simulink model "engine"  (R2019b)
settings: Solver=VariableStepAuto  StartTime=0.0  StopTime=9  MaxStep=1e-2  RelTol=1e-3
libraries: cstblocks x18, simulink x1
(part 2 of 2)

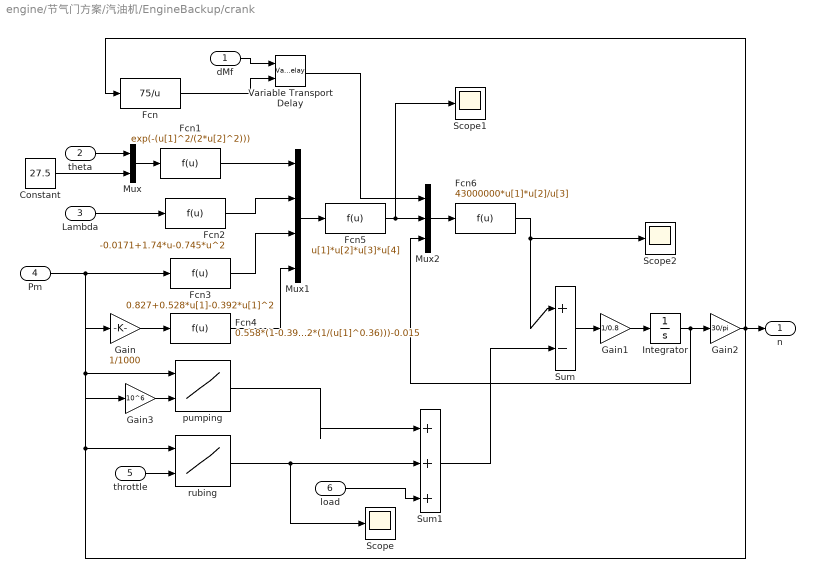
== system engine/节气门方案/汽油机/EngineBackup/crank ==
  dMf : Inport
  theta : Inport  Port=2
  Lambda : Inport  Port=3
  Pm : Inport  Port=4
  throttle : Inport  Port=5
  load : Inport  Port=6
  Constant : Constant  Value=27.5
  Fcn : Fcn  Expr=75/u
  Fcn1 : Fcn  Expr=exp(-(u[1]^2/(2*u[2]^2)))
  Fcn2 : Fcn  Expr=-0.0171+1.74*u-0.745*u^2
  Fcn3 : Fcn  Expr=0.827+0.528*u[1]-0.392*u[1]^2
  Fcn4 : Fcn  Expr=0.558*(1-0.392*(1/(u[1]^0.36)))-0.015
  Fcn5 : Fcn  Expr=u[1]*u[2]*u[3]*u[4]
  Fcn6 : Fcn  Expr=43000000*u[1]*u[2]/u[3]
  Gain : Gain  Gain=1/1000  SaturateOnIntegerOverflow=on  OutDataTypeStr=Inherit: Same as input  ParamDataTypeStr=Inherit: Same as input
  Gain1 : Gain  Gain=1/0.8  SaturateOnIntegerOverflow=on  OutDataTypeStr=Inherit: Same as input  ParamDataTypeStr=Inherit: Same as input
  Gain2 : Gain  Gain=30/pi  SaturateOnIntegerOverflow=on  OutDataTypeStr=Inherit: Same as input  ParamDataTypeStr=Inherit: Same as input
  Gain3 : Gain  Gain=10^6  SaturateOnIntegerOverflow=on  OutDataTypeStr=Inherit: Same as input  ParamDataTypeStr=Inherit: Same as input
  Integrator : Integrator  InitialCondition=349
  Mux : Mux  Inputs=2
  Mux1 : Mux
  Mux2 : Mux  Inputs=3
  Scope : Scope
  Scope1 : Scope
  Scope2 : Scope
  Sum : Sum  Inputs=|+-  SaturateOnIntegerOverflow=on
  Sum1 : Sum  Inputs=|+++  SaturateOnIntegerOverflow=on
  Variable Transport Delay : VariableTransportDelay  MaximumDelay=10
  pumping : Lookup2D  RowIndex=[800 1600 2400 3200 4000 4800 5600 6400]  ColumnIndex=[20000 30000 40000 50000 60000 70000 80000 90000 100000]  Table=[19.6 17.64 15.68 15.68 13.72 11.76 7.84 5.88 3.92;21.56 19.6 17.64 15.68 13.72 11.76 9.8 7.84 3.92;23.52 21.56 19.6 17.64 15.68 13.72 11.76 9.8 7.84;23.52 23.52 19.6 19.6 15.68 15.68 15.68 15.68 13.72;23.52 23.52 23.52 21.56 21.56 21.56 19.6 19.6 19.6;23.52 23.52 23.52 23.52 23.52 25.48 25.48 25.48 25.48;23.52 25.48 25.48 27.44 29.4 31.36 33.32 33.32 35.28;23.52 25.48 27.44 29.4 29.4 31.36 35.28 37.24 39.2]  SaturateOnIntegerOverflow=on
  rubing : Lookup2D  RowIndex=[800 1600 2400 3200 4000 4800 5600 6400]  ColumnIndex=[8 20 32 44 56 68 80 92 104 116]  Table=[31.36 29.4 25.48 23.52 21.56 17.64 15.68 13.72 13.72 13.72;31.36 29.4 25.48 23.52 21.56 17.64 15.68 13.72 13.72 13.72;33.32 29.4 27.44 25.48 21.56 19.6 17.64 15.68 15.68 15.68;33.32 31.36 27.44 25.48 23.52 19.6 17.64 15.68 15.68 15.68;35.28 33.32 29.4 27.44 25.48 21.56 19.6 17.64 17.64 17.64;39.2 37.24 33.32 31.36 29.4 25.48 23.52 21.56 21.56 21.56;45.08 41.16 39.2 37.24 33.32 31.36 29.4 27.44 27.44 27.44;52.92 49 45.08 43.12 41.16 37.24 35.28 33.32 33.32 33.32]  SaturateOnIntegerOverflow=on
  n : Outport
  wires:
  Integrator/1 -> Mux2/3, Gain2/1
  Gain3/1 -> pumping/2
  Sum1/1 -> Sum/2
  load/1 -> Sum1/3
  rubing/1 -> Scope/1, Sum1/2
  pumping/1 -> Sum1/1
  Gain2/1 -> pumping/1, Gain/1, rubing/1, Fcn/1, n/1
  Gain1/1 -> Integrator/1
  Sum/1 -> Gain1/1
  Fcn6/1 -> Scope2/1, Sum/1
  Mux2/1 -> Fcn6/1
  Variable Transport Delay/1 -> Mux2/1
  Fcn5/1 -> Mux2/2, Scope1/1
  Mux1/1 -> Fcn5/1
  throttle/1 -> rubing/2
  Pm/1 -> Fcn3/1, Gain3/1
  Gain/1 -> Fcn4/1
  Fcn4/1 -> Mux1/4
  Fcn3/1 -> Mux1/3
  Fcn2/1 -> Mux1/2
  Fcn1/1 -> Mux1/1
  Lambda/1 -> Fcn2/1
  Mux/1 -> Fcn1/1
  Constant/1 -> Mux/2
  theta/1 -> Mux/1
  Fcn/1 -> Variable Transport Delay/2
  dMf/1 -> Variable Transport Delay/1

== system engine/节气门方案/汽油机/EngineBackup/fuel ==
  a_throttle : Inport
  n : Inport  Port=2
  dMfu : Inport  Port=3
  Subsystem : Subsystem
  Subsystem1 : Subsystem
  dMf : Outport
  wires:
  Subsystem/1(X) -> Subsystem1/2(X)
  Subsystem/2(tau) -> Subsystem1/3(tau)
  Subsystem/3(dMfi) -> Subsystem1/1(dMfi)
  Subsystem1/1(dMf) -> dMf/1
  dMfu/1 -> Subsystem/3(dMfu)
  n/1 -> Subsystem/2(n)
  a_throttle/1 -> Subsystem/1(a_throttle)

== system engine/节气门方案/汽油机/动力输出子模型/摩擦阻力 ==
  Rpm : Inport
  Gain : Gain  Gain=1000
  Sum : Sum  Inputs=|++
  其它机械阻力 : Lookup_n-D  NumberOfTableDimensions=1  BreakpointsForDimension1=[-1000,0,1000,2000,3000,4000,5000,6000,7000]  BreakpointsForDimension2=[1:3]  Table=[-10,0,2.4757,5.0728,8.568,13.3738,18.9078,26.4806,35]  InternalRulePriority=Speed  RndMeth=Simplest  InputSameDT=on
  最大静摩擦 : Saturate  UpperLimit=10  LowerLimit=-10
  摩擦阻力 : Outport
  wires:
  其它机械阻力/1 -> Sum/2
  Sum/1 -> 摩擦阻力/1
  Rpm/1 -> Gain/1, 其它机械阻力/1
  Gain/1 -> 最大静摩擦/1
  最大静摩擦/1 -> Sum/1  "摩擦阻力"

== system engine/节气门方案/汽油机/动力输出子模型/泵气损失 ==
  Pman-kPa : Inport
  rpm : Inport  Port=2
  Lookup::泵气损失 : Lookup_n-D  NumberOfTableDimensions=1  BreakpointsForDimension1=[0,10,20,50,70,90,110,120]  BreakpointsForDimension2=[-250,0,250,500,750,1000,2000,3000,4000,5000,6000,7000]  Table=[99.84,58.6364,37.4242,19.8485,13.1818,9.2424,7.1212,6.5152]  DiagnosticForOutOfRangeInput=Warning  InternalRulePriority=Speed  RndMeth=Simplest  InputSameDT=on
  Product : Product
  泵气损失转速系数 : Gain  Gain=1/1000
  泵气损失 : Outport
  wires:
  rpm/1 -> 泵气损失转速系数/1
  Product/1 -> 泵气损失/1
  Pman-kPa/1 -> Lookup::泵气损失/1
  Lookup::泵气损失/1 -> Product/1
  泵气损失转速系数/1 -> Product/2

== system engine/节气门方案/汽油机/喷油控制、燃油模型/喷油控制算法 ==
  note: dMfv: 需要的燃油蒸汽流量
      | X:燃油喷射沉积比例
  note: dMfu: 通过当前发动机进气量和理论空燃比计算的气缸进油量
  X : Inport
  tau : Inport  Port=2
  dMfu : Inport  Port=3
  Mux : Mux  Inputs=2
  Sum : Sum  Inputs=|+-  SaturateOnIntegerOverflow=on
  由dMfv算dMfi : Fcn  Expr=u[2]/(1-u[1])
  计算油膜蒸发速率:dMff : Subsystem
  dMfi : Outport
  wires:
  计算油膜蒸发速率:dMff/1(dMff) -> Sum/2
  tau/1 -> 计算油膜蒸发速率:dMff/1(tau)
  X/1 -> Mux/1, 计算油膜蒸发速率:dMff/2(X)
  Mux/1 -> 由dMfv算dMfi/1
  由dMfv算dMfi/1 -> 计算油膜蒸发速率:dMff/3(dMfi), dMfi/1  "dMfi"
  Sum/1 -> Mux/2  "dMfv"
  dMfu/1 -> Sum/1

== system engine/节气门方案/汽油机/喷油控制、燃油模型/查表得当前X和tau ==
  throttle : Inport
  n : Inport  Port=2
  Look-Up Table (2-D) : Lookup2D  RowIndex=[0.1 0.2 0.3 0.4 0.5 0.6 0.7 0.8]  ColumnIndex=[1500 2000 2500 3000 4000 5000 6000]  Table=[0.842 0.852 0.852 0.824 0.824 0.842 0.85;0.814 0.847 0.837 0.853 0.85 0.86 0.84;0.838 0.836 0.845 0.856 0.84 0.82 0.86;0.836 0.815 0.865 0.842 0.82 0.87 0.84;0.845 0.824 0.828 0.824 0.85 0.83 0.84;0.841 0.822 0.813 0.832 0.823 0.832 0.845;0.832 0.821 0.841 0.825 0.820 0.832 0.841;0.815 0.808 0.826 0.832 0.815 0.82 0.83]  SaturateOnIntegerOverflow=on
  Look-Up Table (2-D)1 : Lookup2D  RowIndex=[0.1 0.2 0.3 0.4 0.5 0.6 0.7 0.8]  ColumnIndex=[1500 2000 2500 3000 4000 5000 6000]  Table=[0.303 0.238 0.174 0.127 0.125 0.124 0.12;0.335 0.241 0.184 0.131 0.13 0.129 0.12;0.365 0.254 0.195 0.147 0.145 0.125 0.12; 0.374 0.275 0.208 0.152 0.15 0.14 0.13;0.395 0.305 0.216 0.163 0.16 0.15 0.14;0.425 0.336 0.235 0.175 0.170 0.160 0.155;0.438 0.351 0.257 0.182 0.171 0.16 0.54;0.446 0.354 0.262 0.194 0.18 0.175 0.16]  SaturateOnIntegerOverflow=on
  X : Outport
  tau : Outport  Port=2
  wires:
  n/1 -> Look-Up Table (2-D)1/2, Look-Up Table (2-D)/2
  Look-Up Table (2-D)/1 -> X/1
  Look-Up Table (2-D)1/1 -> tau/1
  throttle/1 -> Look-Up Table (2-D)1/1, Look-Up Table (2-D)/1

== system engine/节气门方案/汽油机/喷油控制、燃油模型/燃油模型 ==
  X : Inport
  tau : Inport  Port=2
  dMfi : Inport  Port=3
  1-X : Fcn  Expr=u[1]*(1-u[2])
  1/tau : Math  Operator=reciprocal  SaturateOnIntegerOverflow=on
  Fcn : Fcn  Expr=u[1]*u[2]
  Fcn1 : Fcn  Expr=u[1]*u[2]
  Integrator : Integrator
  Mux : Mux  Inputs=2
  Mux1 : Mux  Inputs=2
  Mux2 : Mux  Inputs=2
  Sum : Sum  Inputs=|++  SaturateOnIntegerOverflow=on
  Sum1 : Sum  Inputs=|+-  SaturateOnIntegerOverflow=on
  X1 : Fcn  Expr=u[1]*u[2]
  dMf : Outport
  wires:
  dMfi/1 -> Mux/1
  X/1 -> Mux/2
  tau/1 -> 1/tau/1
  Sum/1 -> dMf/1
  Fcn1/1 -> Sum1/2
  Mux2/1 -> Fcn1/1
  Integrator/1 -> Sum/2, Mux2/1
  Sum1/1 -> Integrator/1
  Fcn/1 -> Sum1/1
  1-X/1 -> Sum/1
  Mux1/1 -> Fcn/1
  1/tau/1 -> Mux2/2, Mux1/2
  X1/1 -> Mux1/1  "X*dMfi"
  Mux/1 -> X1/1, 1-X/1

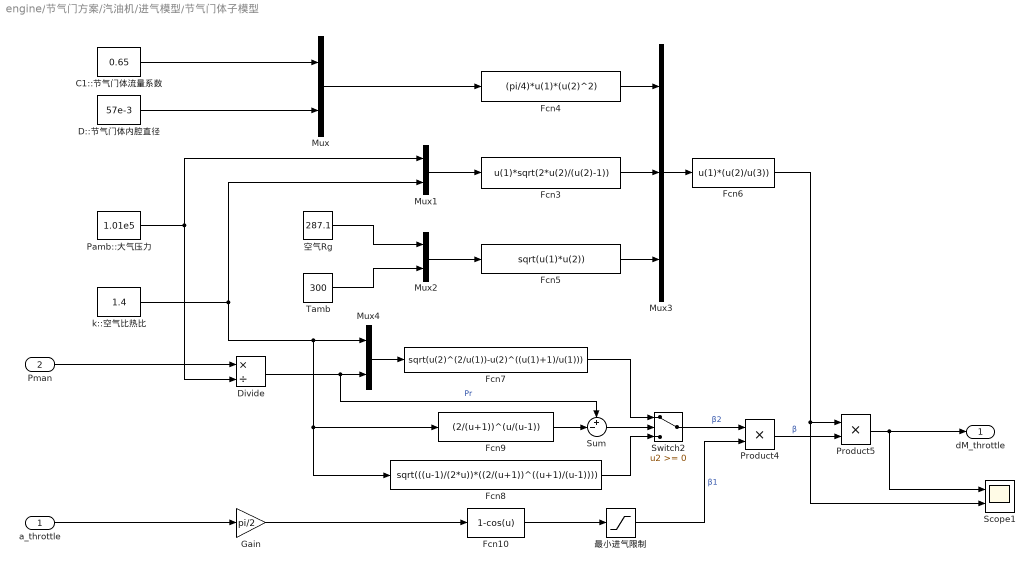
== system engine/节气门方案/汽油机/进气模型/节气门体子模型 ==
  a_throttle : Inport
  Pman : Inport  Port=2
  C1::节气门体流量系数 : Constant  Value=0.65
  D::节气门体内腔直径 : Constant  Value=57e-3
  Divide : Product  Inputs=*/
  Fcn10 : Fcn  Expr=1-cos(u)
  Fcn3 : Fcn  Expr=u(1)*sqrt(2*u(2)/(u(2)-1))
  Fcn4 : Fcn  Expr=(pi/4)*u(1)*(u(2)^2)
  Fcn5 : Fcn  Expr=sqrt(u(1)*u(2))
  Fcn6 : Fcn  Expr=u(1)*(u(2)/u(3))
  Fcn7 : Fcn  Expr=sqrt(u(2)^(2/u(1))-u(2)^((u(1)+1)/u(1)))
  Fcn8 : Fcn  Expr=sqrt(((u-1)/(2*u))*((2/(u+1))^((u+1)/(u-1))))
  Fcn9 : Fcn  Expr=(2/(u+1))^(u/(u-1))
  Gain : Gain  Gain=pi/2
  Mux{,1..2,4} (4 alike) : Mux  Inputs=2
  Mux3 : Mux  Inputs=3
  Pamb::大气压力 : Constant  Value=1.01e5
  Product4 : Product
  Product5 : Product
  Scope1 : Scope  NumInputPorts=2
  Sum : Sum  Inputs=+-|
  Switch2 : Switch  SaturateOnIntegerOverflow=on
  Tamb : Constant  Value=300
  k::空气比热比 : Constant  Value=1.4
  最小进气限制 : Saturate  UpperLimit=1  LowerLimit=0.01
  空气Rg : Constant  Value=287.1
  dM_throttle : Outport
  wires:
  最小进气限制/1 -> Product4/2  "β1"
  Product5/1 -> Scope1/1, dM_throttle/1
  Fcn6/1 -> Product5/1, Scope1/2
  Product4/1 -> Product5/2  "β"
  Gain/1 -> Fcn10/1
  Fcn10/1 -> 最小进气限制/1
  a_throttle/1 -> Gain/1
  Switch2/1 -> Product4/1  "β2"
  Fcn7/1 -> Switch2/1
  Sum/1 -> Switch2/2
  Fcn9/1 -> Sum/2
  Mux4/1 -> Fcn7/1
  Divide/1 -> Mux4/2, Sum/1  "Pr"
  Mux3/1 -> Fcn6/1
  Fcn4/1 -> Mux3/1
  Fcn5/1 -> Mux3/3
  Fcn3/1 -> Mux3/2
  Mux2/1 -> Fcn5/1
  空气Rg/1 -> Mux2/1
  Tamb/1 -> Mux2/2
  Mux1/1 -> Fcn3/1
  k::空气比热比/1 -> Mux4/1, Fcn8/1, Fcn9/1, Mux1/2
  Pamb::大气压力/1 -> Divide/2, Mux1/1
  Mux/1 -> Fcn4/1
  D::节气门体内腔直径/1 -> Mux/2
  C1::节气门体流量系数/1 -> Mux/1
  Fcn8/1 -> Switch2/3
  Pman/1 -> Divide/1

== system engine/节气门方案/汽油机/进气模型/进气歧管子模型 ==
  dM_throttle : Inport
  dM_air_engine : Inport  Port=2
  Gain : Gain  Gain=0.5
  Integrator : Integrator
  Pamb::大气压力 : Constant  Value=1.01e5
  RTm/Vm : Gain  Gain=(287.1*323)/(1.875*(10^(-3)))  SaturateOnIntegerOverflow=on  OutDataTypeStr=Inherit: Same as input  ParamDataTypeStr=Inherit: Same as input
  Sum : Sum  Inputs=|+-  SaturateOnIntegerOverflow=on
  Sum1 : Sum  Inputs=|++
  Pman : Outport
  wires:
  Gain/1 -> Sum1/2
  Pamb::大气压力/1 -> Gain/1
  Sum1/1 -> Pman/1
  dM_throttle/1 -> Sum/1
  dM_air_engine/1 -> Sum/2
  RTm/Vm/1 -> Integrator/1
  Integrator/1 -> Sum1/1
  Sum/1 -> RTm/Vm/1

== system engine/节气门方案/汽油机/进气模型/进气门口模型 ==
  note: Map: 离开进气管，进入燃烧室的空气质量流动速率
  note: Map = n*Vd*η-vol*Pman/(120*R*Tman)
  Pman : Inport
  n : Inport  Port=2
  120R : Gain  Gain=120*287.1  SaturateOnIntegerOverflow=on  OutDataTypeStr=Inherit: Same as input  ParamDataTypeStr=Inherit: Same as input
  Look-Up Table: η-vol : Lookup2D  RowIndex=[40000 50000 65000 80000 90000 95000]  ColumnIndex=[1000 1500 2000 3000 3500 4000 4500 5000]  Table=[0.431 0.5172 0.5532 0.6159 0.5862 0.5847 0.5232 0.4465;0.5705 0.6442 0.6558 0.7246 0.6668 0.6728 0.6235 0.5869;0.6559 0.7401 0.7581 0.7887 0.7638 0.762 0.7321 0.6658;0.7155 0.8231 0.8345 0.8446 0.8279 0.8416 0.8165 0.7365;0.8115 0.8741 0.8636 0.8924 0.8572 0.8752 0.8632 0.8254;0.8621 0.9053 0.9054 0.937 0.904 0.909 0.8865 0.8569]  SaturateOnIntegerOverflow=on
  Product : Product  SaturateOnIntegerOverflow=on  OutDataTypeStr=Inherit: Same as first input
  Product1 : Product  Inputs=***/  SaturateOnIntegerOverflow=on  OutDataTypeStr=Inherit: Same as first input
  Tman : Constant  Value=323
  Vd : Constant  Value=1.5*(10^-3)
  Map : Outport
  wires:
  Pman/1 -> Look-Up Table: η-vol/1, Product/1
  n/1 -> Look-Up Table: η-vol/2, Product/2
  Product/1 -> Product1/1
  Vd/1 -> Product1/2
  Look-Up Table: η-vol/1 -> Product1/3  "η-vol"
  Tman/1 -> 120R/1
  120R/1 -> Product1/4
  Product1/1 -> Map/1  "Map"

== system engine/节气门方案/转速-功率标定/Subsystem1/LPF ==
  Signal : Inport
  Constant2 : Constant  Value=Frq
  Gain : Gain  Gain=2*pi
  d_Smp_LPF6 : cstblocks/Linear Parameter Varying/Varying Lowpass Filter  N=Order
      settings: SourceProductName=Control System Toolbox
  Output : Outport
  wires:
  d_Smp_LPF6/1 -> Output/1  "Is"
  Constant2/1 -> Gain/1
  Signal/1 -> d_Smp_LPF6/1
  Gain/1 -> d_Smp_LPF6/2

== system engine/节气门方案/转速闭环/微分/微分滤波1 ==
  Signal : Inport
  Constant2 : Constant  Value=Frq
  Gain : Gain  Gain=2*pi
  d_Smp_LPF6 : cstblocks/Linear Parameter Varying/Varying Lowpass Filter  N=Order
      settings: SourceProductName=Control System Toolbox
  Output : Outport
  wires:
  d_Smp_LPF6/1 -> Output/1  "Is"
  Constant2/1 -> Gain/1
  Signal/1 -> d_Smp_LPF6/1
  Gain/1 -> d_Smp_LPF6/2

== system engine/节气门方案/转速闭环/积分控制/Subsystem ==
  dErr : Inport
  Err : Inport  Port=2
  Abs : Abs
  Constant10 : Constant
  Constant3 : Constant  Value=0
  Constant4 : Constant
  Memory2 : Memory
  Product : Product
  Switch1 : Switch  Criteria=u2 > Threshold  Threshold=dRPM
  Switch6 : Switch  Criteria=u2 > Threshold
  启动积分 : Outport
  wires:
  Switch1/1 -> 启动积分/1
  Err/1 -> Product/2
  Switch6/1 -> Switch1/1
  Product/1 -> Memory2/1
  Constant3/1 -> Switch6/3
  Abs/1 -> Switch1/2
  Constant4/1 -> Switch1/3
  Constant10/1 -> Switch6/1
  dErr/1 -> Abs/1, Product/1
  Memory2/1 -> Switch6/2

== system engine/节气门方案/转速闭环/积分控制/输出达到正限幅时积分不再增大 ==
  Err : Inport
  Out : Inport  Port=2
  Constant : Constant  Value=Trq_p
  Constant2 : Constant
  Constant5 : Constant  Value=0
  Constant6 : Constant
  Sum2 : Sum  Inputs=-+|
  Switch2 : Switch  Criteria=u2 > Threshold
  Switch3 : Switch  Criteria=u2 > Threshold
  启动积分 : Outport
  wires:
  Err/1 -> Switch2/2
  Switch3/1 -> Switch2/1
  Constant/1 -> Sum2/1
  Constant2/1 -> Switch2/3
  Constant6/1 -> Switch3/3
  Out/1 -> Sum2/2
  Sum2/1 -> Switch3/2
  Switch2/1 -> 启动积分/1
  Constant5/1 -> Switch3/1

== system engine/节气门方案/转速闭环/积分控制/输出达到负限幅时积分不再减小 ==
  Err : Inport
  Out : Inport  Port=2
  Constant1 : Constant
  Constant7 : Constant  Value=0
  Constant8 : Constant
  Constant9 : Constant  Value=-Trq_n
  Sum3 : Sum  Inputs=+-|
  Switch4 : Switch  Criteria=u2 > Threshold
  Switch5 : Switch  Criteria=u2 > Threshold
  启动积分 : Outport
  wires:
  Constant8/1 -> Switch5/3
  Switch4/1 -> 启动积分/1
  Constant7/1 -> Switch5/1
  Constant9/1 -> Sum3/1
  Constant1/1 -> Switch4/1
  Err/1 -> Switch4/2
  Out/1 -> Sum3/2
  Switch5/1 -> Switch4/3
  Sum3/1 -> Switch5/2

== system engine/转速方案/功率闭环/微分/微分滤波1 ==
  Signal : Inport
  Constant2 : Constant  Value=Frq
  Gain : Gain  Gain=2*pi
  d_Smp_LPF6 : cstblocks/Linear Parameter Varying/Varying Lowpass Filter  N=Order
      settings: SourceProductName=Control System Toolbox
  Output : Outport
  wires:
  d_Smp_LPF6/1 -> Output/1  "Is"
  Constant2/1 -> Gain/1
  Signal/1 -> d_Smp_LPF6/1
  Gain/1 -> d_Smp_LPF6/2

== system engine/转速方案/功率闭环/积分控制/Subsystem ==
  dErr : Inport
  Err : Inport  Port=2
  Abs : Abs
  Constant10 : Constant
  Constant3 : Constant  Value=0
  Constant4 : Constant
  Memory2 : Memory
  Product : Product
  Switch1 : Switch  Criteria=u2 > Threshold  Threshold=dPWR
  Switch6 : Switch  Criteria=u2 > Threshold
  启动积分 : Outport
  wires:
  Switch1/1 -> 启动积分/1
  Err/1 -> Product/2
  Switch6/1 -> Switch1/1
  Product/1 -> Memory2/1
  Constant3/1 -> Switch6/3
  Abs/1 -> Switch1/2
  Constant4/1 -> Switch1/3
  Constant10/1 -> Switch6/1
  dErr/1 -> Abs/1, Product/1
  Memory2/1 -> Switch6/2

== system engine/转速方案/功率闭环/积分控制/输出达到正限幅时积分不再增大 ==
  Err : Inport
  Out : Inport  Port=2
  Constant : Constant  Value=Acc_p
  Constant2 : Constant
  Constant5 : Constant  Value=0
  Constant6 : Constant
  Sum2 : Sum  Inputs=-+|
  Switch2 : Switch  Criteria=u2 > Threshold
  Switch3 : Switch  Criteria=u2 > Threshold
  启动积分 : Outport
  wires:
  Err/1 -> Switch2/2
  Switch3/1 -> Switch2/1
  Constant/1 -> Sum2/1
  Constant2/1 -> Switch2/3
  Constant6/1 -> Switch3/3
  Out/1 -> Sum2/2
  Sum2/1 -> Switch3/2
  Switch2/1 -> 启动积分/1
  Constant5/1 -> Switch3/1

== system engine/转速方案/功率闭环/积分控制/输出达到负限幅时积分不再减小 ==
  Err : Inport
  Out : Inport  Port=2
  Constant1 : Constant
  Constant7 : Constant  Value=0
  Constant8 : Constant
  Constant9 : Constant  Value=-Acc_n
  Sum3 : Sum  Inputs=+-|
  Switch4 : Switch  Criteria=u2 > Threshold
  Switch5 : Switch  Criteria=u2 > Threshold
  启动积分 : Outport
  wires:
  Constant8/1 -> Switch5/3
  Switch4/1 -> 启动积分/1
  Constant7/1 -> Switch5/1
  Constant9/1 -> Sum3/1
  Constant1/1 -> Switch4/1
  Err/1 -> Switch4/2
  Out/1 -> Sum3/2
  Switch5/1 -> Switch4/3
  Sum3/1 -> Switch5/2

== system engine/转速方案/汽油机/EngineBackup/air model ==
  n : Inport
  a_throttle : Inport  Port=2
  Gain : Gain  Gain=1/14.7  SaturateOnIntegerOverflow=on  OutDataTypeStr=Inherit: Same as input  ParamDataTypeStr=Inherit: Same as input
  Subsystem : Subsystem
  Subsystem1 : Subsystem
  Subsystem2 : Subsystem
  "dM_air_engine " : Outport
  dMfu : Outport  Port=2
  Pm_pa : Outport  Port=3
  wires:
  n/1 -> Subsystem/2(n)
  Subsystem/1(dM_air_engine) -> "dM_air_engine "/1, Gain/1, Subsystem2/2(dM_air_engine)
  Gain/1 -> dMfu/1
  a_throttle/1 -> Subsystem1/1(a_throttle)
  Subsystem2/1(Pm_pa) -> Pm_pa/1, Subsystem1/2(Pm_pa), Subsystem/1(Pm)
  Subsystem1/1(dM_throttle) -> Subsystem2/1(dM_throttle)

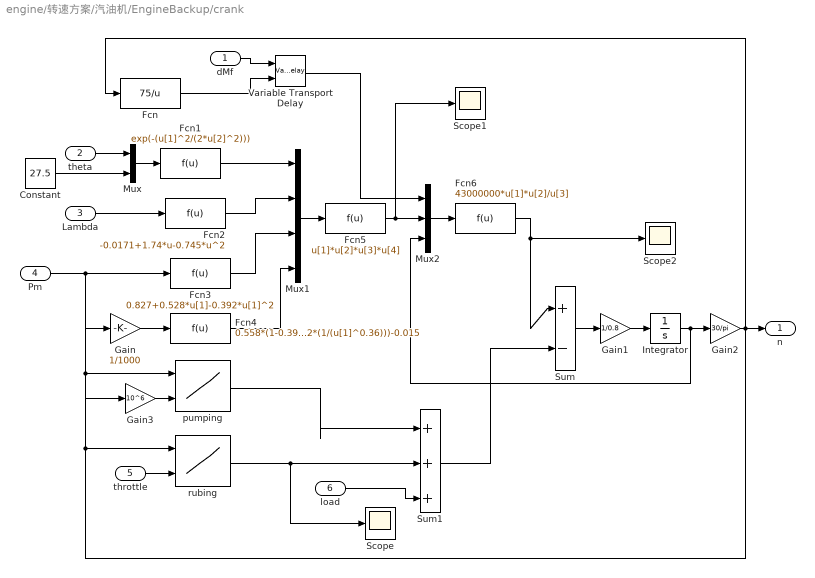
== system engine/转速方案/汽油机/EngineBackup/crank ==
  dMf : Inport
  theta : Inport  Port=2
  Lambda : Inport  Port=3
  Pm : Inport  Port=4
  throttle : Inport  Port=5
  load : Inport  Port=6
  Constant : Constant  Value=27.5
  Fcn : Fcn  Expr=75/u
  Fcn1 : Fcn  Expr=exp(-(u[1]^2/(2*u[2]^2)))
  Fcn2 : Fcn  Expr=-0.0171+1.74*u-0.745*u^2
  Fcn3 : Fcn  Expr=0.827+0.528*u[1]-0.392*u[1]^2
  Fcn4 : Fcn  Expr=0.558*(1-0.392*(1/(u[1]^0.36)))-0.015
  Fcn5 : Fcn  Expr=u[1]*u[2]*u[3]*u[4]
  Fcn6 : Fcn  Expr=43000000*u[1]*u[2]/u[3]
  Gain : Gain  Gain=1/1000  SaturateOnIntegerOverflow=on  OutDataTypeStr=Inherit: Same as input  ParamDataTypeStr=Inherit: Same as input
  Gain1 : Gain  Gain=1/0.8  SaturateOnIntegerOverflow=on  OutDataTypeStr=Inherit: Same as input  ParamDataTypeStr=Inherit: Same as input
  Gain2 : Gain  Gain=30/pi  SaturateOnIntegerOverflow=on  OutDataTypeStr=Inherit: Same as input  ParamDataTypeStr=Inherit: Same as input
  Gain3 : Gain  Gain=10^6  SaturateOnIntegerOverflow=on  OutDataTypeStr=Inherit: Same as input  ParamDataTypeStr=Inherit: Same as input
  Integrator : Integrator  InitialCondition=349
  Mux : Mux  Inputs=2
  Mux1 : Mux
  Mux2 : Mux  Inputs=3
  Scope : Scope
  Scope1 : Scope
  Scope2 : Scope
  Sum : Sum  Inputs=|+-  SaturateOnIntegerOverflow=on
  Sum1 : Sum  Inputs=|+++  SaturateOnIntegerOverflow=on
  Variable Transport Delay : VariableTransportDelay  MaximumDelay=10
  pumping : Lookup2D  RowIndex=[800 1600 2400 3200 4000 4800 5600 6400]  ColumnIndex=[20000 30000 40000 50000 60000 70000 80000 90000 100000]  Table=[19.6 17.64 15.68 15.68 13.72 11.76 7.84 5.88 3.92;21.56 19.6 17.64 15.68 13.72 11.76 9.8 7.84 3.92;23.52 21.56 19.6 17.64 15.68 13.72 11.76 9.8 7.84;23.52 23.52 19.6 19.6 15.68 15.68 15.68 15.68 13.72;23.52 23.52 23.52 21.56 21.56 21.56 19.6 19.6 19.6;23.52 23.52 23.52 23.52 23.52 25.48 25.48 25.48 25.48;23.52 25.48 25.48 27.44 29.4 31.36 33.32 33.32 35.28;23.52 25.48 27.44 29.4 29.4 31.36 35.28 37.24 39.2]  SaturateOnIntegerOverflow=on
  rubing : Lookup2D  RowIndex=[800 1600 2400 3200 4000 4800 5600 6400]  ColumnIndex=[8 20 32 44 56 68 80 92 104 116]  Table=[31.36 29.4 25.48 23.52 21.56 17.64 15.68 13.72 13.72 13.72;31.36 29.4 25.48 23.52 21.56 17.64 15.68 13.72 13.72 13.72;33.32 29.4 27.44 25.48 21.56 19.6 17.64 15.68 15.68 15.68;33.32 31.36 27.44 25.48 23.52 19.6 17.64 15.68 15.68 15.68;35.28 33.32 29.4 27.44 25.48 21.56 19.6 17.64 17.64 17.64;39.2 37.24 33.32 31.36 29.4 25.48 23.52 21.56 21.56 21.56;45.08 41.16 39.2 37.24 33.32 31.36 29.4 27.44 27.44 27.44;52.92 49 45.08 43.12 41.16 37.24 35.28 33.32 33.32 33.32]  SaturateOnIntegerOverflow=on
  n : Outport
  wires:
  dMf/1 -> Variable Transport Delay/1
  Fcn/1 -> Variable Transport Delay/2
  theta/1 -> Mux/1
  Constant/1 -> Mux/2
  Mux/1 -> Fcn1/1
  Lambda/1 -> Fcn2/1
  Fcn1/1 -> Mux1/1
  Fcn2/1 -> Mux1/2
  Fcn3/1 -> Mux1/3
  Fcn4/1 -> Mux1/4
  Gain/1 -> Fcn4/1
  Pm/1 -> Gain3/1, Fcn3/1
  throttle/1 -> rubing/2
  Mux1/1 -> Fcn5/1
  Fcn5/1 -> Scope1/1, Mux2/2
  Variable Transport Delay/1 -> Mux2/1
  Mux2/1 -> Fcn6/1
  Fcn6/1 -> Sum/1, Scope2/1
  Sum/1 -> Gain1/1
  Gain1/1 -> Integrator/1
  Gain2/1 -> n/1, Fcn/1, rubing/1, Gain/1, pumping/1
  pumping/1 -> Sum1/1
  rubing/1 -> Sum1/2, Scope/1
  load/1 -> Sum1/3
  Sum1/1 -> Sum/2
  Gain3/1 -> pumping/2
  Integrator/1 -> Gain2/1, Mux2/3

== system engine/转速方案/汽油机/EngineBackup/fuel ==
  a_throttle : Inport
  n : Inport  Port=2
  dMfu : Inport  Port=3
  Subsystem : Subsystem
  Subsystem1 : Subsystem
  dMf : Outport
  wires:
  a_throttle/1 -> Subsystem/1(a_throttle)
  n/1 -> Subsystem/2(n)
  dMfu/1 -> Subsystem/3(dMfu)
  Subsystem1/1(dMf) -> dMf/1
  Subsystem/3(dMfi) -> Subsystem1/1(dMfi)
  Subsystem/2(tau) -> Subsystem1/3(tau)
  Subsystem/1(X) -> Subsystem1/2(X)

== system engine/转速方案/汽油机/动力输出子模型/摩擦阻力 ==
  Rpm : Inport
  Gain : Gain  Gain=1000
  Sum : Sum  Inputs=|++
  其它机械阻力 : Lookup_n-D  NumberOfTableDimensions=1  BreakpointsForDimension1=[-1000,0,1000,2000,3000,4000,5000,6000,7000]  BreakpointsForDimension2=[1:3]  Table=[-10,0,2.4757,5.0728,8.568,13.3738,18.9078,26.4806,35]  InternalRulePriority=Speed  RndMeth=Simplest  InputSameDT=on
  最大静摩擦 : Saturate  UpperLimit=10  LowerLimit=-10
  摩擦阻力 : Outport
  wires:
  最大静摩擦/1 -> Sum/1  "摩擦阻力"
  Gain/1 -> 最大静摩擦/1
  Rpm/1 -> 其它机械阻力/1, Gain/1
  Sum/1 -> 摩擦阻力/1
  其它机械阻力/1 -> Sum/2

== system engine/转速方案/汽油机/动力输出子模型/泵气损失 ==
  Pman-kPa : Inport
  rpm : Inport  Port=2
  Lookup::泵气损失 : Lookup_n-D  NumberOfTableDimensions=1  BreakpointsForDimension1=[0,10,20,50,70,90,110,120]  BreakpointsForDimension2=[-250,0,250,500,750,1000,2000,3000,4000,5000,6000,7000]  Table=[99.84,58.6364,37.4242,19.8485,13.1818,9.2424,7.1212,6.5152]  DiagnosticForOutOfRangeInput=Warning  InternalRulePriority=Speed  RndMeth=Simplest  InputSameDT=on
  Product : Product
  泵气损失转速系数 : Gain  Gain=1/1000
  泵气损失 : Outport
  wires:
  泵气损失转速系数/1 -> Product/2
  Lookup::泵气损失/1 -> Product/1
  Pman-kPa/1 -> Lookup::泵气损失/1
  Product/1 -> 泵气损失/1
  rpm/1 -> 泵气损失转速系数/1

== system engine/转速方案/汽油机/喷油控制、燃油模型/喷油控制算法 ==
  note: dMfu: 通过当前发动机进气量和理论空燃比计算的气缸进油量
  note: dMfv: 需要的燃油蒸汽流量
      | X:燃油喷射沉积比例
  X : Inport
  tau : Inport  Port=2
  dMfu : Inport  Port=3
  Mux : Mux  Inputs=2
  Sum : Sum  Inputs=|+-  SaturateOnIntegerOverflow=on
  由dMfv算dMfi : Fcn  Expr=u[2]/(1-u[1])
  计算油膜蒸发速率:dMff : Subsystem
  dMfi : Outport
  wires:
  dMfu/1 -> Sum/1
  Sum/1 -> Mux/2  "dMfv"
  由dMfv算dMfi/1 -> dMfi/1, 计算油膜蒸发速率:dMff/3(dMfi)  "dMfi"
  Mux/1 -> 由dMfv算dMfi/1
  X/1 -> 计算油膜蒸发速率:dMff/2(X), Mux/1
  tau/1 -> 计算油膜蒸发速率:dMff/1(tau)
  计算油膜蒸发速率:dMff/1(dMff) -> Sum/2

== system engine/转速方案/汽油机/喷油控制、燃油模型/查表得当前X和tau ==
  throttle : Inport
  n : Inport  Port=2
  Look-Up Table (2-D) : Lookup2D  RowIndex=[0.1 0.2 0.3 0.4 0.5 0.6 0.7 0.8]  ColumnIndex=[1500 2000 2500 3000 4000 5000 6000]  Table=[0.842 0.852 0.852 0.824 0.824 0.842 0.85;0.814 0.847 0.837 0.853 0.85 0.86 0.84;0.838 0.836 0.845 0.856 0.84 0.82 0.86;0.836 0.815 0.865 0.842 0.82 0.87 0.84;0.845 0.824 0.828 0.824 0.85 0.83 0.84;0.841 0.822 0.813 0.832 0.823 0.832 0.845;0.832 0.821 0.841 0.825 0.820 0.832 0.841;0.815 0.808 0.826 0.832 0.815 0.82 0.83]  SaturateOnIntegerOverflow=on
  Look-Up Table (2-D)1 : Lookup2D  RowIndex=[0.1 0.2 0.3 0.4 0.5 0.6 0.7 0.8]  ColumnIndex=[1500 2000 2500 3000 4000 5000 6000]  Table=[0.303 0.238 0.174 0.127 0.125 0.124 0.12;0.335 0.241 0.184 0.131 0.13 0.129 0.12;0.365 0.254 0.195 0.147 0.145 0.125 0.12; 0.374 0.275 0.208 0.152 0.15 0.14 0.13;0.395 0.305 0.216 0.163 0.16 0.15 0.14;0.425 0.336 0.235 0.175 0.170 0.160 0.155;0.438 0.351 0.257 0.182 0.171 0.16 0.54;0.446 0.354 0.262 0.194 0.18 0.175 0.16]  SaturateOnIntegerOverflow=on
  X : Outport
  tau : Outport  Port=2
  wires:
  throttle/1 -> Look-Up Table (2-D)/1, Look-Up Table (2-D)1/1
  Look-Up Table (2-D)1/1 -> tau/1
  Look-Up Table (2-D)/1 -> X/1
  n/1 -> Look-Up Table (2-D)/2, Look-Up Table (2-D)1/2

== system engine/转速方案/汽油机/喷油控制、燃油模型/燃油模型 ==
  X : Inport
  tau : Inport  Port=2
  dMfi : Inport  Port=3
  1-X : Fcn  Expr=u[1]*(1-u[2])
  1/tau : Math  Operator=reciprocal  SaturateOnIntegerOverflow=on
  Fcn : Fcn  Expr=u[1]*u[2]
  Fcn1 : Fcn  Expr=u[1]*u[2]
  Integrator : Integrator
  Mux : Mux  Inputs=2
  Mux1 : Mux  Inputs=2
  Mux2 : Mux  Inputs=2
  Sum : Sum  Inputs=|++  SaturateOnIntegerOverflow=on
  Sum1 : Sum  Inputs=|+-  SaturateOnIntegerOverflow=on
  X1 : Fcn  Expr=u[1]*u[2]
  dMf : Outport
  wires:
  Mux/1 -> 1-X/1, X1/1
  X1/1 -> Mux1/1  "X*dMfi"
  1/tau/1 -> Mux1/2, Mux2/2
  Mux1/1 -> Fcn/1
  1-X/1 -> Sum/1
  Fcn/1 -> Sum1/1
  Sum1/1 -> Integrator/1
  Integrator/1 -> Mux2/1, Sum/2
  Mux2/1 -> Fcn1/1
  Fcn1/1 -> Sum1/2
  Sum/1 -> dMf/1
  tau/1 -> 1/tau/1
  X/1 -> Mux/2
  dMfi/1 -> Mux/1

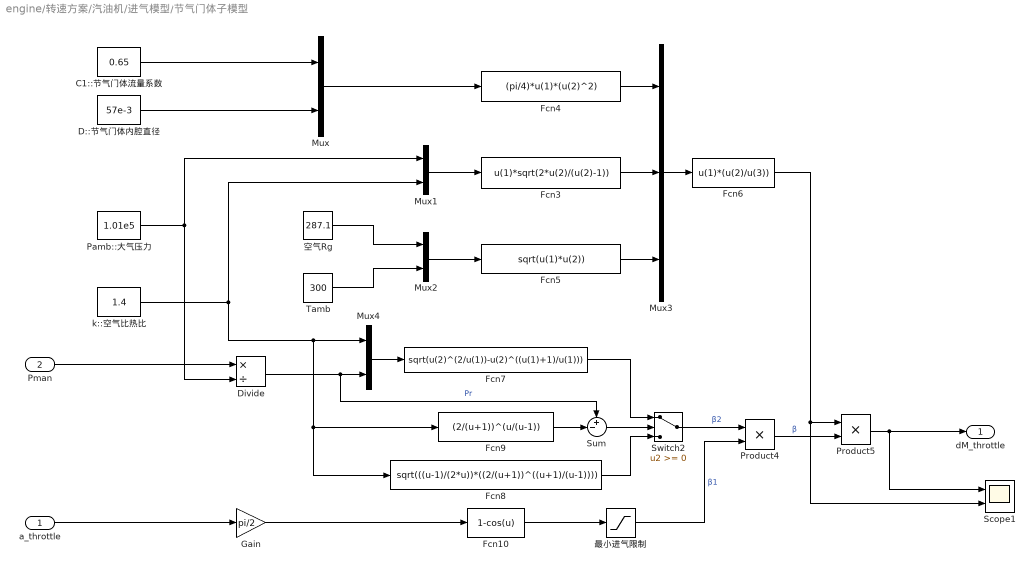
== system engine/转速方案/汽油机/进气模型/节气门体子模型 ==
  a_throttle : Inport
  Pman : Inport  Port=2
  C1::节气门体流量系数 : Constant  Value=0.65
  D::节气门体内腔直径 : Constant  Value=57e-3
  Divide : Product  Inputs=*/
  Fcn10 : Fcn  Expr=1-cos(u)
  Fcn3 : Fcn  Expr=u(1)*sqrt(2*u(2)/(u(2)-1))
  Fcn4 : Fcn  Expr=(pi/4)*u(1)*(u(2)^2)
  Fcn5 : Fcn  Expr=sqrt(u(1)*u(2))
  Fcn6 : Fcn  Expr=u(1)*(u(2)/u(3))
  Fcn7 : Fcn  Expr=sqrt(u(2)^(2/u(1))-u(2)^((u(1)+1)/u(1)))
  Fcn8 : Fcn  Expr=sqrt(((u-1)/(2*u))*((2/(u+1))^((u+1)/(u-1))))
  Fcn9 : Fcn  Expr=(2/(u+1))^(u/(u-1))
  Gain : Gain  Gain=pi/2
  Mux{,1..2,4} (4 alike) : Mux  Inputs=2
  Mux3 : Mux  Inputs=3
  Pamb::大气压力 : Constant  Value=1.01e5
  Product4 : Product
  Product5 : Product
  Scope1 : Scope  NumInputPorts=2
  Sum : Sum  Inputs=+-|
  Switch2 : Switch  SaturateOnIntegerOverflow=on
  Tamb : Constant  Value=300
  k::空气比热比 : Constant  Value=1.4
  最小进气限制 : Saturate  UpperLimit=1  LowerLimit=0.02
  空气Rg : Constant  Value=287.1
  dM_throttle : Outport
  wires:
  Pman/1 -> Divide/1
  Fcn8/1 -> Switch2/3
  C1::节气门体流量系数/1 -> Mux/1
  D::节气门体内腔直径/1 -> Mux/2
  Mux/1 -> Fcn4/1
  Pamb::大气压力/1 -> Mux1/1, Divide/2
  k::空气比热比/1 -> Mux1/2, Fcn9/1, Fcn8/1, Mux4/1
  Mux1/1 -> Fcn3/1
  Tamb/1 -> Mux2/2
  空气Rg/1 -> Mux2/1
  Mux2/1 -> Fcn5/1
  Fcn3/1 -> Mux3/2
  Fcn5/1 -> Mux3/3
  Fcn4/1 -> Mux3/1
  Mux3/1 -> Fcn6/1
  Divide/1 -> Sum/1, Mux4/2  "Pr"
  Mux4/1 -> Fcn7/1
  Fcn9/1 -> Sum/2
  Sum/1 -> Switch2/2
  Fcn7/1 -> Switch2/1
  Switch2/1 -> Product4/1  "β2"
  a_throttle/1 -> Gain/1
  Fcn10/1 -> 最小进气限制/1
  Gain/1 -> Fcn10/1
  Product4/1 -> Product5/2  "β"
  Fcn6/1 -> Scope1/2, Product5/1
  Product5/1 -> dM_throttle/1, Scope1/1
  最小进气限制/1 -> Product4/2  "β1"

== system engine/转速方案/汽油机/进气模型/进气歧管子模型 ==
  dM_throttle : Inport
  dM_air_engine : Inport  Port=2
  Gain : Gain  Gain=0.5
  Integrator : Integrator
  Pamb::大气压力 : Constant  Value=1.01e5
  RTm/Vm : Gain  Gain=(287.1*323)/(1.875*(10^(-3)))  SaturateOnIntegerOverflow=on  OutDataTypeStr=Inherit: Same as input  ParamDataTypeStr=Inherit: Same as input
  Sum : Sum  Inputs=|+-  SaturateOnIntegerOverflow=on
  Sum1 : Sum  Inputs=|++
  Pman : Outport
  wires:
  Sum/1 -> RTm/Vm/1
  Integrator/1 -> Sum1/1
  RTm/Vm/1 -> Integrator/1
  dM_air_engine/1 -> Sum/2
  dM_throttle/1 -> Sum/1
  Sum1/1 -> Pman/1
  Pamb::大气压力/1 -> Gain/1
  Gain/1 -> Sum1/2

== system engine/转速方案/汽油机/进气模型/进气门口模型 ==
  note: Map = n*Vd*η-vol*Pman/(120*R*Tman)
  note: Map: 离开进气管，进入燃烧室的空气质量流动速率
  Pman : Inport
  n : Inport  Port=2
  120R : Gain  Gain=120*287.1  SaturateOnIntegerOverflow=on  OutDataTypeStr=Inherit: Same as input  ParamDataTypeStr=Inherit: Same as input
  Look-Up Table: η-vol : Lookup2D  RowIndex=[40000 50000 65000 80000 90000 95000]  ColumnIndex=[1000 1500 2000 3000 3500 4000 4500 5000]  Table=[0.431 0.5172 0.5532 0.6159 0.5862 0.5847 0.5232 0.4465;0.5705 0.6442 0.6558 0.7246 0.6668 0.6728 0.6235 0.5869;0.6559 0.7401 0.7581 0.7887 0.7638 0.762 0.7321 0.6658;0.7155 0.8231 0.8345 0.8446 0.8279 0.8416 0.8165 0.7365;0.8115 0.8741 0.8636 0.8924 0.8572 0.8752 0.8632 0.8254;0.8621 0.9053 0.9054 0.937 0.904 0.909 0.8865 0.8569]  SaturateOnIntegerOverflow=on
  Product : Product  SaturateOnIntegerOverflow=on  OutDataTypeStr=Inherit: Same as first input
  Product1 : Product  Inputs=***/  SaturateOnIntegerOverflow=on  OutDataTypeStr=Inherit: Same as first input
  Tman : Constant  Value=323
  Vd : Constant  Value=1.5*(10^-3)
  Map : Outport
  wires:
  Product1/1 -> Map/1  "Map"
  120R/1 -> Product1/4
  Tman/1 -> 120R/1
  Look-Up Table: η-vol/1 -> Product1/3  "η-vol"
  Vd/1 -> Product1/2
  Product/1 -> Product1/1
  n/1 -> Product/2, Look-Up Table: η-vol/2
  Pman/1 -> Product/1, Look-Up Table: η-vol/1

== system engine/转速方案/油门信号控制/转速稳定检查/转速反馈滤波 ==
  Signal : Inport
  Constant2 : Constant  Value=Frq
  Gain : Gain  Gain=2*pi
  d_Smp_LPF6 : cstblocks/Linear Parameter Varying/Varying Lowpass Filter  N=Order
      settings: SourceProductName=Control System Toolbox
  Output : Outport
  wires:
  d_Smp_LPF6/1 -> Output/1  "Is"
  Constant2/1 -> Gain/1
  Signal/1 -> d_Smp_LPF6/1
  Gain/1 -> d_Smp_LPF6/2

== system engine/转速方案/转速闭环/微分/微分滤波1 ==
  Signal : Inport
  Constant2 : Constant  Value=Frq
  Gain : Gain  Gain=2*pi
  d_Smp_LPF6 : cstblocks/Linear Parameter Varying/Varying Lowpass Filter  N=Order
      settings: SourceProductName=Control System Toolbox
  Output : Outport
  wires:
  Gain/1 -> d_Smp_LPF6/2
  Signal/1 -> d_Smp_LPF6/1
  Constant2/1 -> Gain/1
  d_Smp_LPF6/1 -> Output/1  "Is"

== system engine/转速方案/转速闭环/积分控制/Subsystem ==
  dErr : Inport
  Err : Inport  Port=2
  Abs : Abs
  Constant10 : Constant
  Constant3 : Constant  Value=0
  Constant4 : Constant
  Memory2 : Memory
  Product : Product
  Switch1 : Switch  Criteria=u2 > Threshold  Threshold=dRPM
  Switch6 : Switch  Criteria=u2 > Threshold
  启动积分 : Outport
  wires:
  Memory2/1 -> Switch6/2
  dErr/1 -> Product/1, Abs/1
  Constant10/1 -> Switch6/1
  Constant4/1 -> Switch1/3
  Abs/1 -> Switch1/2
  Constant3/1 -> Switch6/3
  Product/1 -> Memory2/1
  Switch6/1 -> Switch1/1
  Err/1 -> Product/2
  Switch1/1 -> 启动积分/1

== system engine/转速方案/转速闭环/积分控制/输出达到正限幅时积分不再增大 ==
  Err : Inport
  Out : Inport  Port=2
  Constant : Constant  Value=Trq_p
  Constant2 : Constant
  Constant5 : Constant  Value=0
  Constant6 : Constant
  Sum2 : Sum  Inputs=-+|
  Switch2 : Switch  Criteria=u2 > Threshold
  Switch3 : Switch  Criteria=u2 > Threshold
  启动积分 : Outport
  wires:
  Constant5/1 -> Switch3/1
  Switch2/1 -> 启动积分/1
  Sum2/1 -> Switch3/2
  Out/1 -> Sum2/2
  Constant6/1 -> Switch3/3
  Constant2/1 -> Switch2/3
  Constant/1 -> Sum2/1
  Switch3/1 -> Switch2/1
  Err/1 -> Switch2/2

== system engine/转速方案/转速闭环/积分控制/输出达到负限幅时积分不再减小 ==
  Err : Inport
  Out : Inport  Port=2
  Constant1 : Constant
  Constant7 : Constant  Value=0
  Constant8 : Constant
  Constant9 : Constant  Value=-Trq_n
  Sum3 : Sum  Inputs=+-|
  Switch4 : Switch  Criteria=u2 > Threshold
  Switch5 : Switch  Criteria=u2 > Threshold
  启动积分 : Outport
  wires:
  Sum3/1 -> Switch5/2
  Switch5/1 -> Switch4/3
  Out/1 -> Sum3/2
  Err/1 -> Switch4/2
  Constant1/1 -> Switch4/1
  Constant9/1 -> Sum3/1
  Constant7/1 -> Switch5/1
  Switch4/1 -> 启动积分/1
  Constant8/1 -> Switch5/3

== system engine/节气门方案/汽油机/EngineBackup/air model/Subsystem ==
  Pm : Inport
  n : Inport  Port=2
  120R : Gain  Gain=120*287.1  SaturateOnIntegerOverflow=on  OutDataTypeStr=Inherit: Same as input  ParamDataTypeStr=Inherit: Same as input
  Constant : Constant  Value=1.5*(10^-3)
  Constant1 : Constant  Value=323
  Look-Up Table (2-D) : Lookup2D  RowIndex=[50000 60000 70000 80000 90000 95000]  ColumnIndex=[1500 2000 2500 3000 3500 4000 4500 5000]  Table=[0.431 0.5172 0.5532 0.6159 0.5862 0.5847 0.5232 0.4465;0.5705 0.6442 0.6558 0.7246 0.6668 0.6728 0.6235 0.5869;0.6559 0.7401 0.7581 0.7887 0.7638 0.762 0.7321 0.6658;0.7155 0.8231 0.8345 0.8446 0.8279 0.8416 0.8165 0.7365;0.8115 0.8741 0.8636 0.8924 0.8572 0.8752 0.8632 0.8254;0.8621 0.9053 0.9054 0.937 0.904 0.909 0.8865 0.8569]  SaturateOnIntegerOverflow=on
  Product : Product  SaturateOnIntegerOverflow=on  OutDataTypeStr=Inherit: Same as first input
  Product1 : Product  Inputs=***/  SaturateOnIntegerOverflow=on  OutDataTypeStr=Inherit: Same as first input
  dM_air_engine : Outport
  wires:
  Product1/1 -> dM_air_engine/1
  120R/1 -> Product1/4
  Constant1/1 -> 120R/1
  Look-Up Table (2-D)/1 -> Product1/3
  Constant/1 -> Product1/2
  Product/1 -> Product1/1
  n/1 -> Product/2, Look-Up Table (2-D)/2
  Pm/1 -> Product/1, Look-Up Table (2-D)/1

== system engine/节气门方案/汽油机/EngineBackup/air model/Subsystem1 ==
  a_throttle : Inport
  Pm_pa : Inport  Port=2
  Constant : Constant  Value=287.1
  Constant1 : Constant  Value=300
  Constant2 : Constant  Value=0.6848
  Fcn : Fcn  Expr=2.388*u+4.4146
  Fcn1 : Fcn  Expr=-31.329*u^4+27.2*u^3-2.0028*u^2+6.7647*u-0.10775
  Fcn2 : Fcn  Expr=sqrt(7*(u^(2/1.4)-u^(2.4/1.4)))
  Gain1 : Gain  Gain=10^-4  SaturateOnIntegerOverflow=on  OutDataTypeStr=Inherit: Same as input  ParamDataTypeStr=Inherit: Same as input
  Math Function : Math  Operator=sqrt  SaturateOnIntegerOverflow=on
  Pa : Constant  Value=0.989*10^5
  Product : Product  Inputs=*/  SaturateOnIntegerOverflow=on  OutDataTypeStr=Inherit: Same as first input
  Product1 : Product  SaturateOnIntegerOverflow=on  OutDataTypeStr=Inherit: Same as first input
  Product2 : Product  Inputs=*/  SaturateOnIntegerOverflow=on  OutDataTypeStr=Inherit: Same as first input
  Product3 : Product  Inputs=3  SaturateOnIntegerOverflow=on  OutDataTypeStr=Inherit: Same as first input
  Switch : Switch  Threshold=0.85  SaturateOnIntegerOverflow=on
  Switch1 : Switch  Threshold=0.5283  SaturateOnIntegerOverflow=on
  dM_throttle : Outport
  wires:
  Product3/1 -> dM_throttle/1
  Product2/1 -> Product3/3
  Switch1/1 -> Product3/2
  Gain1/1 -> Product3/1
  Switch/1 -> Gain1/1
  Constant2/1 -> Switch1/3
  Fcn2/1 -> Switch1/1
  Product/1 -> Switch1/2, Fcn2/1
  Math Function/1 -> Product2/2
  Product1/1 -> Math Function/1
  Constant1/1 -> Product1/2
  Constant/1 -> Product1/1
  Pa/1 -> Product2/1, Product/2
  Pm_pa/1 -> Product/1
  Fcn1/1 -> Switch/3
  Fcn/1 -> Switch/1
  a_throttle/1 -> Fcn1/1, Fcn/1, Switch/2

== system engine/节气门方案/汽油机/EngineBackup/air model/Subsystem2 ==
  dM_throttle : Inport
  dM_air_engine : Inport  Port=2
  Integrator : Integrator
  RTm/Vm : Gain  Gain=(287.1*323)/(1.875*(10^(-3)))  SaturateOnIntegerOverflow=on  OutDataTypeStr=Inherit: Same as input  ParamDataTypeStr=Inherit: Same as input
  Sum : Sum  Inputs=|+-  SaturateOnIntegerOverflow=on
  Pm_pa : Outport
  wires:
  Sum/1 -> RTm/Vm/1
  Integrator/1 -> Pm_pa/1
  RTm/Vm/1 -> Integrator/1
  dM_air_engine/1 -> Sum/2
  dM_throttle/1 -> Sum/1

== system engine/节气门方案/汽油机/EngineBackup/fuel/Subsystem ==
  a_throttle : Inport
  n : Inport  Port=2
  dMfu : Inport  Port=3
  Fcn : Fcn  Expr=u[2]/(1-u[1])
  Fcn1 : Fcn  Expr=u[1]*u[2]
  Fcn2 : Fcn  Expr=u[1]*u[2]*u[3]
  Integrator : Integrator
  Look-Up Table (2-D) : Lookup2D  RowIndex=[0.1 0.2 0.3 0.4 0.5 0.6 0.7 0.8]  ColumnIndex=[1500 2000 2500 3000 4000 5000 6000]  Table=[0.842 0.852 0.852 0.824 0.824 0.842 0.85;0.814 0.847 0.837 0.853 0.85 0.86 0.84;0.838 0.836 0.845 0.856 0.84 0.82 0.86;0.836 0.815 0.865 0.842 0.82 0.87 0.84;0.845 0.824 0.828 0.824 0.85 0.83 0.84;0.841 0.822 0.813 0.832 0.823 0.832 0.845;0.832 0.821 0.841 0.825 0.820 0.832 0.841;0.815 0.808 0.826 0.832 0.815 0.82 0.83]  SaturateOnIntegerOverflow=on
  Look-Up Table (2-D)1 : Lookup2D  RowIndex=[0.1 0.2 0.3 0.4 0.5 0.6 0.7 0.8]  ColumnIndex=[1500 2000 2500 3000 4000 5000 6000]  Table=[0.303 0.238 0.174 0.127 0.125 0.124 0.12;0.335 0.241 0.184 0.131 0.13 0.129 0.12;0.365 0.254 0.195 0.147 0.145 0.125 0.12; 0.374 0.275 0.208 0.152 0.15 0.14 0.13;0.395 0.305 0.216 0.163 0.16 0.15 0.14;0.425 0.336 0.235 0.175 0.170 0.160 0.155;0.438 0.351 0.257 0.182 0.171 0.16 0.54;0.446 0.354 0.262 0.194 0.18 0.175 0.16]  SaturateOnIntegerOverflow=on
  Math Function : Math  Operator=reciprocal  SaturateOnIntegerOverflow=on
  Mux : Mux  Inputs=2
  Mux1 : Mux  Inputs=3
  Mux2 : Mux  Inputs=2
  Sum : Sum  Inputs=|+-  SaturateOnIntegerOverflow=on
  Sum1 : Sum  Inputs=-+  SaturateOnIntegerOverflow=on
  X : Outport
  tau : Outport  Port=2
  dMfi : Outport  Port=3
  wires:
  Fcn2/1 -> Sum1/2
  Mux1/1 -> Fcn2/1
  Fcn1/1 -> Sum1/1
  Sum1/1 -> Integrator/1
  Integrator/1 -> Mux2/1, Sum/2
  Mux2/1 -> Fcn1/1
  Fcn/1 -> dMfi/1, Mux1/3
  Math Function/1 -> Mux2/2, Mux1/2
  Mux/1 -> Fcn/1
  Sum/1 -> Mux/2
  dMfu/1 -> Sum/1
  Look-Up Table (2-D)/1 -> X/1, Mux/1, Mux1/1
  Look-Up Table (2-D)1/1 -> tau/1, Math Function/1
  n/1 -> Look-Up Table (2-D)/2, Look-Up Table (2-D)1/2
  a_throttle/1 -> Look-Up Table (2-D)/1, Look-Up Table (2-D)1/1

== system engine/节气门方案/汽油机/EngineBackup/fuel/Subsystem1 ==
  dMfi : Inport
  X : Inport  Port=2
  tau : Inport  Port=3
  1-X : Fcn  Expr=u[1]*(1-u[2])
  1/tau : Math  Operator=reciprocal  SaturateOnIntegerOverflow=on
  Fcn : Fcn  Expr=u[1]*u[2]
  Fcn1 : Fcn  Expr=u[1]*u[2]
  Integrator : Integrator
  Mux : Mux  Inputs=2
  Mux1 : Mux  Inputs=2
  Mux2 : Mux  Inputs=2
  Sum : Sum  Inputs=|++  SaturateOnIntegerOverflow=on
  Sum1 : Sum  Inputs=|+-  SaturateOnIntegerOverflow=on
  X1 : Fcn  Expr=u[1]*u[2]
  dMf : Outport
  wires:
  Mux/1 -> X1/1, 1-X/1
  X1/1 -> Mux1/1
  1/tau/1 -> Mux2/2, Mux1/2
  Mux1/1 -> Fcn/1
  1-X/1 -> Sum/1
  Fcn/1 -> Sum1/1
  Sum1/1 -> Integrator/1
  Integrator/1 -> Mux2/1, Sum/2
  Mux2/1 -> Fcn1/1
  Fcn1/1 -> Sum1/2
  Sum/1 -> dMf/1
  tau/1 -> 1/tau/1
  X/1 -> Mux/2
  dMfi/1 -> Mux/1

== system engine/节气门方案/汽油机/喷油控制、燃油模型/喷油控制算法/计算油膜蒸发速率:dMff ==
  note: 注：求解微分方程，收敛得到dMff
  tau : Inport
  X : Inport  Port=2
  dMfi : Inport  Port=3
  Fcn1 : Fcn  Expr=u[1]*u[2]
  Fcn2 : Fcn  Expr=u[1]*u[2]*u[3]
  Integrator : Integrator
  Math Function : Math  Operator=reciprocal  SaturateOnIntegerOverflow=on
  Mux1 : Mux  Inputs=3
  Mux2 : Mux  Inputs=2
  Sum1 : Sum  Inputs=-+  SaturateOnIntegerOverflow=on
  dMff : Outport
  wires:
  X/1 -> Mux1/2
  dMfi/1 -> Mux1/3
  Mux2/1 -> Fcn1/1
  Math Function/1 -> Mux1/1, Mux2/2  "1/tau"
  Sum1/1 -> Integrator/1  "ddMff"
  tau/1 -> Math Function/1
  Mux1/1 -> Fcn2/1
  Integrator/1 -> dMff/1, Mux2/1
  Fcn1/1 -> Sum1/1  "dMff/tau"
  Fcn2/1 -> Sum1/2

== system engine/转速方案/汽油机/EngineBackup/air model/Subsystem ==
  Pm : Inport
  n : Inport  Port=2
  120R : Gain  Gain=120*287.1  SaturateOnIntegerOverflow=on  OutDataTypeStr=Inherit: Same as input  ParamDataTypeStr=Inherit: Same as input
  Constant : Constant  Value=1.5*(10^-3)
  Constant1 : Constant  Value=323
  Look-Up Table (2-D) : Lookup2D  RowIndex=[50000 60000 70000 80000 90000 95000]  ColumnIndex=[1500 2000 2500 3000 3500 4000 4500 5000]  Table=[0.431 0.5172 0.5532 0.6159 0.5862 0.5847 0.5232 0.4465;0.5705 0.6442 0.6558 0.7246 0.6668 0.6728 0.6235 0.5869;0.6559 0.7401 0.7581 0.7887 0.7638 0.762 0.7321 0.6658;0.7155 0.8231 0.8345 0.8446 0.8279 0.8416 0.8165 0.7365;0.8115 0.8741 0.8636 0.8924 0.8572 0.8752 0.8632 0.8254;0.8621 0.9053 0.9054 0.937 0.904 0.909 0.8865 0.8569]  SaturateOnIntegerOverflow=on
  Product : Product  SaturateOnIntegerOverflow=on  OutDataTypeStr=Inherit: Same as first input
  Product1 : Product  Inputs=***/  SaturateOnIntegerOverflow=on  OutDataTypeStr=Inherit: Same as first input
  dM_air_engine : Outport
  wires:
  Pm/1 -> Look-Up Table (2-D)/1, Product/1
  n/1 -> Look-Up Table (2-D)/2, Product/2
  Product/1 -> Product1/1
  Constant/1 -> Product1/2
  Look-Up Table (2-D)/1 -> Product1/3
  Constant1/1 -> 120R/1
  120R/1 -> Product1/4
  Product1/1 -> dM_air_engine/1

== system engine/转速方案/汽油机/EngineBackup/air model/Subsystem1 ==
  a_throttle : Inport
  Pm_pa : Inport  Port=2
  Constant : Constant  Value=287.1
  Constant1 : Constant  Value=300
  Constant2 : Constant  Value=0.6848
  Fcn : Fcn  Expr=2.388*u+4.4146
  Fcn1 : Fcn  Expr=-31.329*u^4+27.2*u^3-2.0028*u^2+6.7647*u-0.10775
  Fcn2 : Fcn  Expr=sqrt(7*(u^(2/1.4)-u^(2.4/1.4)))
  Gain1 : Gain  Gain=10^-4  SaturateOnIntegerOverflow=on  OutDataTypeStr=Inherit: Same as input  ParamDataTypeStr=Inherit: Same as input
  Math Function : Math  Operator=sqrt  SaturateOnIntegerOverflow=on
  Pa : Constant  Value=0.989*10^5
  Product : Product  Inputs=*/  SaturateOnIntegerOverflow=on  OutDataTypeStr=Inherit: Same as first input
  Product1 : Product  SaturateOnIntegerOverflow=on  OutDataTypeStr=Inherit: Same as first input
  Product2 : Product  Inputs=*/  SaturateOnIntegerOverflow=on  OutDataTypeStr=Inherit: Same as first input
  Product3 : Product  Inputs=3  SaturateOnIntegerOverflow=on  OutDataTypeStr=Inherit: Same as first input
  Switch : Switch  Threshold=0.85  SaturateOnIntegerOverflow=on
  Switch1 : Switch  Threshold=0.5283  SaturateOnIntegerOverflow=on
  dM_throttle : Outport
  wires:
  a_throttle/1 -> Switch/2, Fcn/1, Fcn1/1
  Fcn/1 -> Switch/1
  Fcn1/1 -> Switch/3
  Pm_pa/1 -> Product/1
  Pa/1 -> Product/2, Product2/1
  Constant/1 -> Product1/1
  Constant1/1 -> Product1/2
  Product1/1 -> Math Function/1
  Math Function/1 -> Product2/2
  Product/1 -> Fcn2/1, Switch1/2
  Fcn2/1 -> Switch1/1
  Constant2/1 -> Switch1/3
  Switch/1 -> Gain1/1
  Gain1/1 -> Product3/1
  Switch1/1 -> Product3/2
  Product2/1 -> Product3/3
  Product3/1 -> dM_throttle/1

== system engine/转速方案/汽油机/EngineBackup/air model/Subsystem2 ==
  dM_throttle : Inport
  dM_air_engine : Inport  Port=2
  Integrator : Integrator
  RTm/Vm : Gain  Gain=(287.1*323)/(1.875*(10^(-3)))  SaturateOnIntegerOverflow=on  OutDataTypeStr=Inherit: Same as input  ParamDataTypeStr=Inherit: Same as input
  Sum : Sum  Inputs=|+-  SaturateOnIntegerOverflow=on
  Pm_pa : Outport
  wires:
  dM_throttle/1 -> Sum/1
  dM_air_engine/1 -> Sum/2
  RTm/Vm/1 -> Integrator/1
  Integrator/1 -> Pm_pa/1
  Sum/1 -> RTm/Vm/1

== system engine/转速方案/汽油机/EngineBackup/fuel/Subsystem ==
  a_throttle : Inport
  n : Inport  Port=2
  dMfu : Inport  Port=3
  Fcn : Fcn  Expr=u[2]/(1-u[1])
  Fcn1 : Fcn  Expr=u[1]*u[2]
  Fcn2 : Fcn  Expr=u[1]*u[2]*u[3]
  Integrator : Integrator
  Look-Up Table (2-D) : Lookup2D  RowIndex=[0.1 0.2 0.3 0.4 0.5 0.6 0.7 0.8]  ColumnIndex=[1500 2000 2500 3000 4000 5000 6000]  Table=[0.842 0.852 0.852 0.824 0.824 0.842 0.85;0.814 0.847 0.837 0.853 0.85 0.86 0.84;0.838 0.836 0.845 0.856 0.84 0.82 0.86;0.836 0.815 0.865 0.842 0.82 0.87 0.84;0.845 0.824 0.828 0.824 0.85 0.83 0.84;0.841 0.822 0.813 0.832 0.823 0.832 0.845;0.832 0.821 0.841 0.825 0.820 0.832 0.841;0.815 0.808 0.826 0.832 0.815 0.82 0.83]  SaturateOnIntegerOverflow=on
  Look-Up Table (2-D)1 : Lookup2D  RowIndex=[0.1 0.2 0.3 0.4 0.5 0.6 0.7 0.8]  ColumnIndex=[1500 2000 2500 3000 4000 5000 6000]  Table=[0.303 0.238 0.174 0.127 0.125 0.124 0.12;0.335 0.241 0.184 0.131 0.13 0.129 0.12;0.365 0.254 0.195 0.147 0.145 0.125 0.12; 0.374 0.275 0.208 0.152 0.15 0.14 0.13;0.395 0.305 0.216 0.163 0.16 0.15 0.14;0.425 0.336 0.235 0.175 0.170 0.160 0.155;0.438 0.351 0.257 0.182 0.171 0.16 0.54;0.446 0.354 0.262 0.194 0.18 0.175 0.16]  SaturateOnIntegerOverflow=on
  Math Function : Math  Operator=reciprocal  SaturateOnIntegerOverflow=on
  Mux : Mux  Inputs=2
  Mux1 : Mux  Inputs=3
  Mux2 : Mux  Inputs=2
  Sum : Sum  Inputs=|+-  SaturateOnIntegerOverflow=on
  Sum1 : Sum  Inputs=-+  SaturateOnIntegerOverflow=on
  X : Outport
  tau : Outport  Port=2
  dMfi : Outport  Port=3
  wires:
  a_throttle/1 -> Look-Up Table (2-D)1/1, Look-Up Table (2-D)/1
  n/1 -> Look-Up Table (2-D)1/2, Look-Up Table (2-D)/2
  Look-Up Table (2-D)1/1 -> Math Function/1, tau/1
  Look-Up Table (2-D)/1 -> Mux1/1, Mux/1, X/1
  dMfu/1 -> Sum/1
  Sum/1 -> Mux/2
  Mux/1 -> Fcn/1
  Math Function/1 -> Mux1/2, Mux2/2
  Fcn/1 -> Mux1/3, dMfi/1
  Mux2/1 -> Fcn1/1
  Integrator/1 -> Sum/2, Mux2/1
  Sum1/1 -> Integrator/1
  Fcn1/1 -> Sum1/1
  Mux1/1 -> Fcn2/1
  Fcn2/1 -> Sum1/2

== system engine/转速方案/汽油机/EngineBackup/fuel/Subsystem1 ==
  dMfi : Inport
  X : Inport  Port=2
  tau : Inport  Port=3
  1-X : Fcn  Expr=u[1]*(1-u[2])
  1/tau : Math  Operator=reciprocal  SaturateOnIntegerOverflow=on
  Fcn : Fcn  Expr=u[1]*u[2]
  Fcn1 : Fcn  Expr=u[1]*u[2]
  Integrator : Integrator
  Mux : Mux  Inputs=2
  Mux1 : Mux  Inputs=2
  Mux2 : Mux  Inputs=2
  Sum : Sum  Inputs=|++  SaturateOnIntegerOverflow=on
  Sum1 : Sum  Inputs=|+-  SaturateOnIntegerOverflow=on
  X1 : Fcn  Expr=u[1]*u[2]
  dMf : Outport
  wires:
  dMfi/1 -> Mux/1
  X/1 -> Mux/2
  tau/1 -> 1/tau/1
  Sum/1 -> dMf/1
  Fcn1/1 -> Sum1/2
  Mux2/1 -> Fcn1/1
  Integrator/1 -> Sum/2, Mux2/1
  Sum1/1 -> Integrator/1
  Fcn/1 -> Sum1/1
  1-X/1 -> Sum/1
  Mux1/1 -> Fcn/1
  1/tau/1 -> Mux1/2, Mux2/2
  X1/1 -> Mux1/1
  Mux/1 -> 1-X/1, X1/1

== system engine/转速方案/汽油机/喷油控制、燃油模型/喷油控制算法/计算油膜蒸发速率:dMff ==
  note: 注：求解微分方程，收敛得到dMff
  tau : Inport
  X : Inport  Port=2
  dMfi : Inport  Port=3
  Fcn1 : Fcn  Expr=u[1]*u[2]
  Fcn2 : Fcn  Expr=u[1]*u[2]*u[3]
  Integrator : Integrator
  Math Function : Math  Operator=reciprocal  SaturateOnIntegerOverflow=on
  Mux1 : Mux  Inputs=3
  Mux2 : Mux  Inputs=2
  Sum1 : Sum  Inputs=-+  SaturateOnIntegerOverflow=on
  dMff : Outport
  wires:
  Fcn2/1 -> Sum1/2
  Fcn1/1 -> Sum1/1  "dMff/tau"
  Integrator/1 -> Mux2/1, dMff/1
  Mux1/1 -> Fcn2/1
  tau/1 -> Math Function/1
  Sum1/1 -> Integrator/1  "ddMff"
  Math Function/1 -> Mux2/2, Mux1/1  "1/tau"
  Mux2/1 -> Fcn1/1
  dMfi/1 -> Mux1/3
  X/1 -> Mux1/2
